simulink model "powerfrompropagatorLoLaSat"  (R2023b)
settings: Solver=FixedStepAuto  StartTime=0.0  StopTime=t_sim  FixedStep=TimeStep  RelTol=1e-3
undefined symbols (not defined in the file or in its folder): angle_roll, date, juliandate, MODE, Psa_X, Psa_Y, PsaX, PsaY
libraries: dspmathops x16, vrlib x12, aerolibutil x9, sharedtransform x9, sharedutil x4
settings Model: Creator=colpari  LastModifiedBy=lricc
settings SolverCC: AlgebraicLoopSolver=TrustRegion
settings OptimizationCC: ReuseModelBlockBuffer=off
settings DebuggingCC: UnconnectedInputMsg=warning  UnconnectedOutputMsg=warning  UnconnectedLineMsg=warning
settings ModelReferenceCC: EnableRefExpFcnMdlSchedulingChecks=on
settings RTWCC: DLArmComputeVersion=19.05

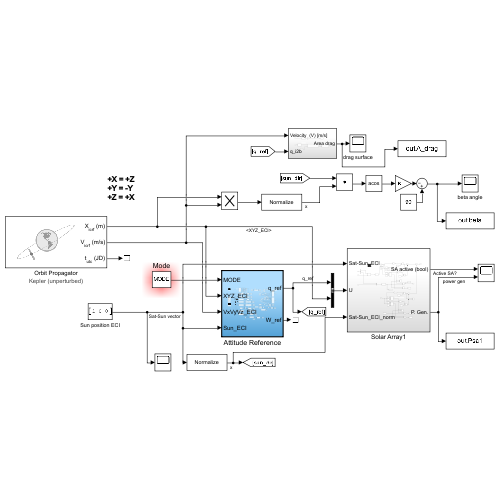
[thumbnail: Simulink's stored preview of the top-level diagram]
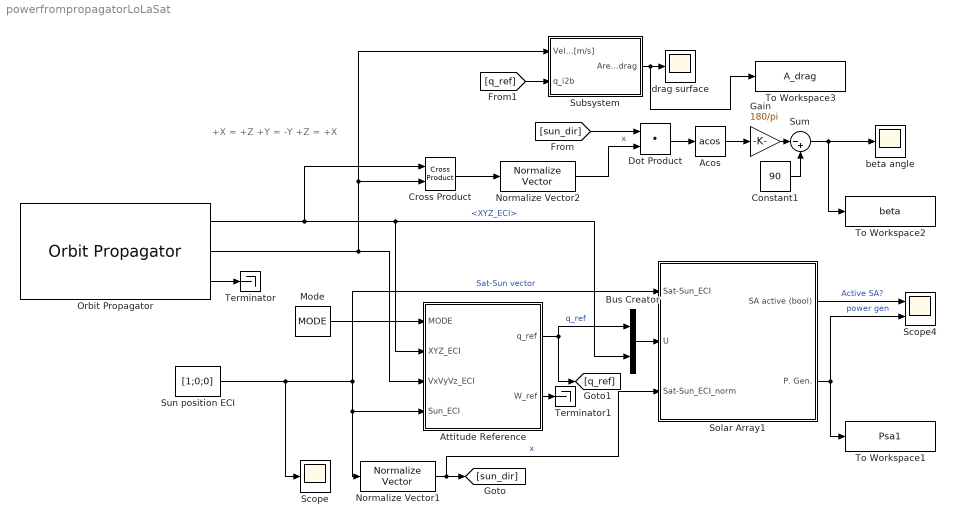
== system powerfrompropagatorLoLaSat ==
  note: +X = +Z
      | +Y = -Y
      | +Z = +X
  Acos : Trigonometry  Operator=acos
  Attitude Reference : Subsystem  TreatAsAtomicUnit=on
  Bus Creator : BusCreator  Inputs=2
  Constant1 : Constant  Value=90
  Cross Product : vrlib/Utilities/Cross Product
  Dot Product : DotProduct  OutDataTypeStr=Inherit: Inherit via internal rule
  Gain : Gain  Gain=180/pi
  Mode : Constant  Value=MODE  OutDataTypeStr=int8
  Normalize Vector1 : vrlib/Utilities/Normalize Vector  maxzero=0
  Normalize Vector2 : vrlib/Utilities/Normalize Vector  maxzero=0
  Orbit Propagator : OrbitPropagator  startDate=juliandate(date.year, date.month, date.day, date.hour, date.minutes, date.seconds)  semiMajorAxis=orbit.a  eccentricity=orbit.e  inclination=orbit.i  raan=orbit.O  argPeriapsis=orbit.o  trueAnomaly=orbit.nu  inertialPosition=[3649700.0 3308200.0 -4676600.0]  inertialVelocity=[-2750.8 6666.4 2573.4]  fixedPosition=[-4142689.0 -2676864.7 -4669861.6]  fixedVelocity=[1452.7 -6720.7 2568.1]  customR=3396200  customMu=4.305e13  customJ2=1.0826269e-03  customOmega=4.06125949e-3
      settings: AttributesFormatString=%<propagator>
  Scope : Scope
  Scope4 : Scope  NumInputPorts=2
  Solar Array1 : Subsystem
  Subsystem : Subsystem
  Sum : Sum  Inputs=|-+
  Sun position ECI : Constant  Value=[1;0;0]
  Terminator : Terminator
  Terminator1 : Terminator
  To Workspace1 : ToWorkspace  VariableName=Psa1  SaveFormat=Timeseries  SampleTime=-1
  To Workspace2 : ToWorkspace  VariableName=beta  SaveFormat=Timeseries  SampleTime=-1
  To Workspace3 : ToWorkspace  VariableName=A_drag  SaveFormat=Timeseries  SampleTime=-1
  beta angle : Scope
  drag surface : Scope
  wires:
  Dot Product/1 -> Acos/1
  Attitude Reference/1(q_ref) -> [q_ref], Bus Creator/1  "q_ref"
  Sum/1 -> beta angle/1, To Workspace2/1
  Cross Product/1 -> Normalize Vector2/1
  Solar Array1/2(P. Gen.) -> To Workspace1/1, Scope4/2  "power gen"
  [sun_dir] -> Dot Product/1
  Acos/1 -> Gain/1
  Orbit Propagator/2 -> Attitude Reference/3(VxVyVz_ECI), Subsystem/1(Velocity  (V) [m/s]), Cross Product/2
  Gain/1 -> Sum/1
  Sun position ECI/1 -> Scope/1, Solar Array1/1(Sat-Sun_ECI), Attitude Reference/4(Sun_ECI), Normalize Vector1/1  "Sat-Sun vector"
  Constant1/1 -> Sum/2
  Normalize Vector1/1 -> Solar Array1/3(Sat-Sun_ECI_norm), [sun_dir]  "x"
  Bus Creator/1 -> Solar Array1/2(U)
  Normalize Vector2/1 -> Dot Product/2  "x"
  Solar Array1/1(SA active (bool)) -> Scope4/1  "Active SA?"
  Orbit Propagator/1 -> Attitude Reference/2(XYZ_ECI), Bus Creator/2, Cross Product/1  "<XYZ_ECI>"
  Orbit Propagator/3 -> Terminator/1
  Attitude Reference/2(W_ref) -> Terminator1/1
  Mode/1 -> Attitude Reference/1(MODE)
  [q_ref] -> Subsystem/2(q_i2b)
  Subsystem/1(Area drag) -> To Workspace3/1, drag surface/1

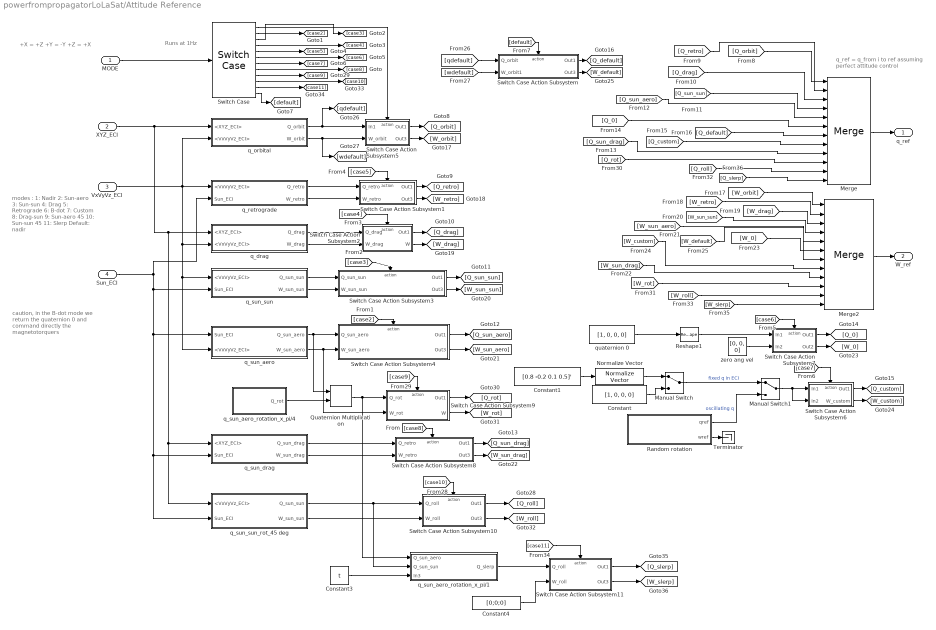
== system powerfrompropagatorLoLaSat/Attitude Reference ==
  note: caution, in the B-dot mode we return the quaternion 0 and command directly the magnetotorquers
  note: modes :
      | 1: Nadir
      | 2: Sun-aero
      | 3: Sun-sun
      | 4: Drag
      | 5: Retrograde
      | 6: B-dot
      | 7: Custom
      | 8: Drag-sun
      | 9: Sun-aero 45
      | 10: Sun-sun 45
      | 11: Slerp
      | Default: nadir
  note: q_ref  = q_from i to ref
      | assuming perfect attitude control
  note: Runs at 1Hz
  note: +X = +Z
      | +Y = -Y
      | +Z = +X
  MODE : Inport  OutMin=1  OutMax=100  OutDataTypeStr=int8
  XYZ_ECI : Inport  Port=2
  VxVyVz_ECI : Inport  Port=3
  Sun_ECI : Inport  Port=4
  Constant : Constant  Value=[1, 0, 0, 0]
  Constant1 : Constant  Value=[0.8 -0.2 0.1 0.5]'
  Constant3 : Constant  Value=t
  Constant4 : Constant  Value=[0;0;0]
  Manual Switch : ManualSwitch
  Manual Switch1 : ManualSwitch
  Merge : Merge  Inputs=12
  Merge2 : Merge  Inputs=12
  Normalize Vector : vrlib/Utilities/Normalize Vector  maxzero=0
  Quaternion Multiplication : aerolibutil/Quaternion Multiplication
  Random rotation : Subsystem
  Reshape1 : Reshape  OutputDimensionality=Column vector (2-D)
  Switch Case : SwitchCase  CaseConditions={1, 2, 3, 4, 5, 6, 7, 8, 9, 10, 11}
  Switch Case Action Subsystem : Subsystem  TreatAsAtomicUnit=on
  Switch Case Action Subsystem1 : Subsystem  TreatAsAtomicUnit=on
  Switch Case Action Subsystem10 : Subsystem  TreatAsAtomicUnit=on
  Switch Case Action Subsystem11 : Subsystem  TreatAsAtomicUnit=on
  Switch Case Action Subsystem2 : Subsystem  TreatAsAtomicUnit=on
  Switch Case Action Subsystem3 : Subsystem  TreatAsAtomicUnit=on
  Switch Case Action Subsystem4 : Subsystem  TreatAsAtomicUnit=on
  Switch Case Action Subsystem5 : Subsystem  TreatAsAtomicUnit=on
  Switch Case Action Subsystem6 : Subsystem  TreatAsAtomicUnit=on
  Switch Case Action Subsystem7 : Subsystem  TreatAsAtomicUnit=on
  Switch Case Action Subsystem8 : Subsystem  TreatAsAtomicUnit=on
  Switch Case Action Subsystem9 : Subsystem  TreatAsAtomicUnit=on
  Terminator : Terminator
  q_drag : Subsystem
  q_orbital : Subsystem
  q_retrograde : Subsystem
  q_sun_aero : Subsystem
  q_sun_aero_rotation_x_pi/1 : Subsystem
  q_sun_aero_rotation_x_pi/4 : Subsystem
  q_sun_drag : Subsystem
  q_sun_sun : Subsystem
  q_sun_sun_rot_45 deg : Subsystem
  quaternion 0 : Constant  Value=[1, 0, 0, 0]
  zero ang vel : Constant  Value=[0, 0, 0]
  q_ref : Outport  VectorParamsAs1DForOutWhenUnconnected=off
  W_ref : Outport  Port=2
  wires:
  quaternion 0/1 -> Reshape1/1
  Reshape1/1 -> Switch Case Action Subsystem7/1(In1)
  Constant/1 -> Manual Switch/2
  Constant1/1 -> Normalize Vector/1
  Normalize Vector/1 -> Manual Switch/1
  zero ang vel/1 -> Switch Case Action Subsystem7/2(In2)
  Manual Switch/1 -> Manual Switch1/1  "fixed q in ECI"
  Random rotation/1(qref) -> Manual Switch1/2  "oscillating q"
  Manual Switch1/1 -> Switch Case Action Subsystem6/2(In2), Switch Case Action Subsystem6/1(In1)
  [default] -> Switch Case Action Subsystem/Action
  Switch Case/7 -> [case7]
  Switch Case/4 -> [case4]
  Switch Case/5 -> [case5]
  [case3] -> Switch Case Action Subsystem3/Action
  [case5] -> Switch Case Action Subsystem1/Action
  Switch Case/3 -> [case3]
  Switch Case/2 -> [case2]
  q_drag/2(W_drag) -> Switch Case Action Subsystem2/2(W_drag)
  q_sun_drag/2(W_sun_drag) -> Switch Case Action Subsystem8/2(W_retro)
  q_sun_aero/2(W_sun_aero) -> Switch Case Action Subsystem9/2(W_rot), Switch Case Action Subsystem4/2(W_sun_aero)
  Switch Case/1 -> Switch Case Action Subsystem5/Action
  [case8] -> Switch Case Action Subsystem8/Action
  Switch Case/8 -> [case8]
  q_drag/1(Q_drag) -> Switch Case Action Subsystem2/1(Q_drag)
  Switch Case/12 -> [default]
  q_sun_sun/2(W_sun_sun) -> Switch Case Action Subsystem3/2(W_sun_sun)
  q_retrograde/2(W_retro) -> Switch Case Action Subsystem1/2(W_retro)
  q_sun_sun/1(Q_sun_sun) -> Switch Case Action Subsystem3/1(Q_sun_sun)
  q_sun_aero/1(Q_sun_aero) -> Quaternion Multiplication/1, Switch Case Action Subsystem4/1(Q_sun_aero)
  q_sun_drag/1(Q_sun_drag) -> Switch Case Action Subsystem8/1(Q_retro)
  Merge2/1 -> W_ref/1
  [case2] -> Switch Case Action Subsystem4/Action
  [case4] -> Switch Case Action Subsystem2/Action
  q_orbital/1(Q_orbit) -> [qdefault], Switch Case Action Subsystem5/1(In1)
  q_retrograde/1(Q_retro) -> Switch Case Action Subsystem1/1(Q_retro)
  q_orbital/2(W_orbit) -> [wdefault], Switch Case Action Subsystem5/2(W_orbit)
  Switch Case/6 -> [case6]
  VxVyVz_ECI/1 -> q_orbital/2(<VxVyVz_ECI>), q_retrograde/1(<VxVyVz_ECI>), q_drag/2(<VxVyVz_ECI>), q_sun_aero/2(<VxVyVz_ECI>), q_sun_sun/1(<VxVyVz_ECI>)
  Merge/1 -> q_ref/1
  MODE/1 -> Switch Case/1
  Random rotation/2(wref) -> Terminator/1
  [case6] -> Switch Case Action Subsystem7/Action
  [case7] -> Switch Case Action Subsystem6/Action
  Switch Case Action Subsystem5/1(Out1) -> [Q_orbit]
  [Q_orbit] -> Merge/1
  Switch Case Action Subsystem1/1(Out1) -> [Q_retro]
  [Q_retro] -> Merge/2
  Switch Case Action Subsystem2/1(Out1) -> [Q_drag]
  [Q_drag] -> Merge/3
  Switch Case Action Subsystem3/1(Out1) -> [Q_sun_sun]
  [Q_sun_sun] -> Merge/4
  Switch Case Action Subsystem4/1(Out1) -> [Q_sun_aero]
  [Q_sun_aero] -> Merge/5
  Switch Case Action Subsystem8/1(Out1) -> [Q_sun_drag]
  [Q_sun_drag] -> Merge/9
  Switch Case Action Subsystem7/1(Out1) -> [Q_0]
  [Q_0] -> Merge/6
  Switch Case Action Subsystem6/1(Out1) -> [Q_custom]
  [Q_custom] -> Merge/8
  Switch Case Action Subsystem/1(Out1) -> [Q_default]
  [Q_default] -> Merge/7
  Switch Case Action Subsystem5/2(Out3) -> [W_orbit]
  [W_orbit] -> Merge2/1
  Switch Case Action Subsystem1/2(Out3) -> [W_retro]
  [W_retro] -> Merge2/2
  Switch Case Action Subsystem2/2(W) -> [W_drag]
  [W_drag] -> Merge2/3
  Switch Case Action Subsystem3/2(Out3) -> [W_sun_sun]
  [W_sun_sun] -> Merge2/4
  Switch Case Action Subsystem4/2(Out3) -> [W_sun_aero]
  [W_sun_aero] -> Merge2/5
  Switch Case Action Subsystem8/2(Out3) -> [W_sun_drag]
  [W_sun_drag] -> Merge2/9
  Switch Case Action Subsystem7/2(Out2) -> [W_0]
  [W_0] -> Merge2/6
  Switch Case Action Subsystem6/2(W_custom) -> [W_custom]
  [W_custom] -> Merge2/8
  Switch Case Action Subsystem/2(Out3) -> [W_default]
  [W_default] -> Merge2/7
  [qdefault] -> Switch Case Action Subsystem/1(Q_orbit)
  [wdefault] -> Switch Case Action Subsystem/2(W_orbit1)
  q_sun_aero_rotation_x_pi/4/1(Q_rot) -> Quaternion Multiplication/2
  Quaternion Multiplication/1 -> q_sun_aero_rotation_x_pi/1/1(Q_sun_aero), Switch Case Action Subsystem9/1(Q_rot)
  Switch Case/9 -> [case9]
  [case9] -> Switch Case Action Subsystem9/Action
  Switch Case Action Subsystem9/1(Out1) -> [Q_rot]
  Switch Case Action Subsystem9/2(W) -> [W_rot]
  [Q_rot] -> Merge/10
  [W_rot] -> Merge2/10
  Sun_ECI/1 -> q_retrograde/2(Sun_ECI), q_sun_sun_rot_45 deg/2(Sun_ECI), q_sun_drag/2(Sun_ECI), q_sun_aero/1(Sun_ECI), q_sun_sun/2(Sun_ECI)
  q_sun_sun_rot_45 deg/1(Q_sun_sun) -> q_sun_aero_rotation_x_pi/1/2(Q_sun_sun), Switch Case Action Subsystem10/1(Q_roll)
  XYZ_ECI/1 -> q_sun_drag/1(<XYZ_ECI>), q_sun_sun_rot_45 deg/1(<VxVyVz_ECI>), q_drag/1(<XYZ_ECI>), q_orbital/1(<XYZ_ECI>)
  Switch Case Action Subsystem10/1(Out1) -> [Q_roll]
  [case10] -> Switch Case Action Subsystem10/Action
  q_sun_sun_rot_45 deg/2(W_sun_sun) -> Switch Case Action Subsystem10/2(W_roll)
  Switch Case Action Subsystem10/2(Out3) -> [W_roll]
  Switch Case/10 -> [case10]
  [Q_roll] -> Merge/11
  [W_roll] -> Merge2/11
  Switch Case/11 -> [case11]
  [W_slerp] -> Merge2/12
  Constant3/1 -> q_sun_aero_rotation_x_pi/1/3(In3)
  Switch Case Action Subsystem11/2(Out3) -> [W_slerp]
  [case11] -> Switch Case Action Subsystem11/Action
  Switch Case Action Subsystem11/1(Out1) -> [Q_slerp]
  q_sun_aero_rotation_x_pi/1/1(Q_slerp) -> Switch Case Action Subsystem11/1(Q_roll)
  Constant4/1 -> Switch Case Action Subsystem11/2(W_roll)
  [Q_slerp] -> Merge/12

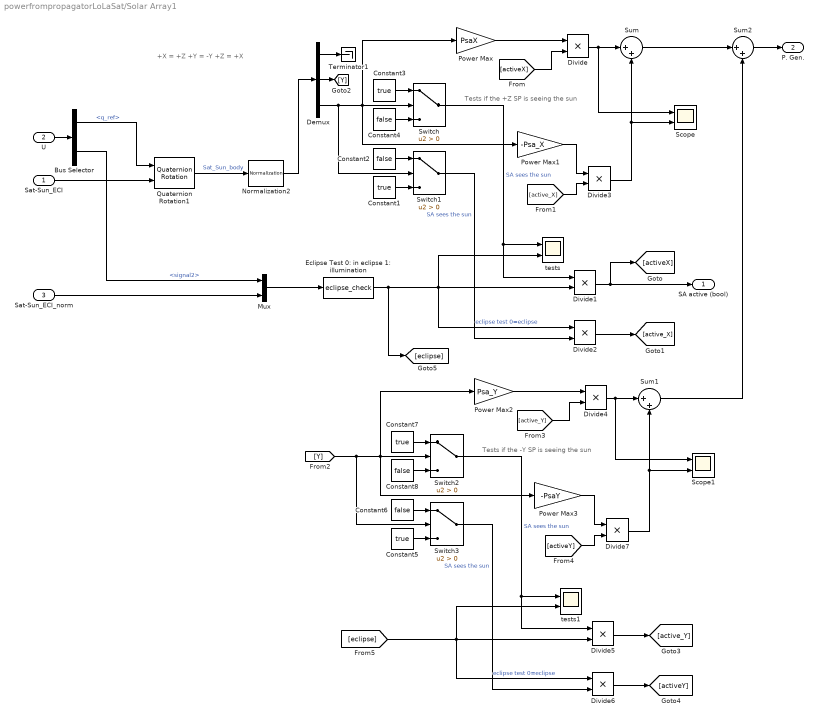
== system powerfrompropagatorLoLaSat/Solar Array1 ==
  note: Tests if the +Z SP is seeing the sun
  note: +X = +Z
      | +Y = -Y
      | +Z = +X
  note: Tests if the -Y SP is seeing the sun
  Sat-Sun_ECI : Inport
  U : Inport  Port=2
  Sat-Sun_ECI_norm : Inport  Port=3
  Bus Selector : BusSelector  OutputSignals=q_ref,signal2
  Constant{1,3,5,7} (4 alike) : Constant  Value=true
  Constant{2,4,6,8} (4 alike) : Constant  Value=false
  Demux : Demux  Outputs=3
  Divide{,1..7} (8 alike) : Product  Inputs=**
  Eclipse Test 0: in eclipse 1: illumination : MATLABFcn  MATLABFcn=eclipse_check
  Mux : Mux  Inputs=2
  Normalization2 : dspmathops/Normalization  NormType=2-norm  Bias=1e-10  NormOver=Each column  Dimension=1  roundingMode=Floor  overflowMode=off  accumDataTypeStr=Inherit: Same as product output  accumLastDataTypeStr=Inherit: Same as product output  outputDataTypeStr=Inherit: Same as product output  outputMin=[]  outputMax=[]  outputLastDataTypeStr=Inherit: Same as product output
  Power Max : Gain  Gain=PsaX
  Power Max1 : Gain  Gain=-Psa_X
  Power Max2 : Gain  Gain=Psa_Y
  Power Max3 : Gain  Gain=-PsaY
  Quaternion Rotation1 : aerolibutil/Quaternion Rotation
  Scope : Scope  NumInputPorts=2
  Scope1 : Scope  NumInputPorts=2
  Sum : Sum  Inputs=|++
  Sum1 : Sum  Inputs=|++
  Sum2 : Sum  Inputs=|++
  Switch{,1..3} (4 alike) : Switch  Criteria=u2 > Threshold  SaturateOnIntegerOverflow=off  InputSameDT=off
  Terminator1 : Terminator
  tests : Scope  NumInputPorts=2
  tests1 : Scope  NumInputPorts=2
  SA active (bool) : Outport  VectorParamsAs1DForOutWhenUnconnected=off
  P. Gen. : Outport  Port=2
  wires:
  Switch/1 -> Divide1/1, tests/1  "SA sees the sun"
  U/1 -> Bus Selector/1
  Bus Selector/1 -> Quaternion Rotation1/1  "<q_ref>"
  Quaternion Rotation1/1 -> Normalization2/1  "Sat_Sun_body"
  Constant3/1 -> Switch/1
  Demux/2 -> [Y]
  Demux/1 -> Terminator1/1
  Bus Selector/2 -> Mux/1  "<signal2>"
  Divide1/1 -> [activeX], SA active (bool)/1
  Constant4/1 -> Switch/3
  Normalization2/1 -> Demux/1
  Divide/1 -> Scope/1, Sum/1
  Power Max/1 -> Divide/1
  [activeX] -> Divide/2
  Sat-Sun_ECI_norm/1 -> Mux/2
  Mux/1 -> Eclipse Test 0: in eclipse 1: illumination/1
  Eclipse Test 0: in eclipse 1: illumination/1 -> [eclipse], Divide2/1, tests/2, Divide1/2  "eclipse test 0=eclipse"
  Demux/3 -> Switch1/2, Power Max1/1, Power Max/1, Switch/2
  Constant2/1 -> Switch1/1
  Constant1/1 -> Switch1/3
  Switch1/1 -> Divide2/2  "SA sees the sun"
  Divide2/1 -> [active_X]
  [active_X] -> Divide3/2
  Power Max1/1 -> Divide3/1
  Divide3/1 -> Sum/2, Scope/2
  Sum/1 -> Sum2/1
  [Y] -> Switch3/2, Power Max3/1, Power Max2/1, Switch2/2
  [eclipse] -> Divide6/1, tests1/2, Divide5/2  "eclipse test 0=eclipse"
  [active_Y] -> Divide4/2
  Constant7/1 -> Switch2/1
  Divide5/1 -> [active_Y]
  Constant8/1 -> Switch2/3
  Switch2/1 -> Divide5/1, tests1/1  "SA sees the sun"
  Sum1/1 -> Sum2/2
  Divide6/1 -> [activeY]
  Divide4/1 -> Scope1/1, Sum1/1
  Switch3/1 -> Divide6/2  "SA sees the sun"
  Constant6/1 -> Switch3/1
  Power Max2/1 -> Divide4/1
  [activeY] -> Divide7/2
  Power Max3/1 -> Divide7/1
  Divide7/1 -> Scope1/2, Sum1/2
  Constant5/1 -> Switch3/3
  Sum2/1 -> P. Gen./1
  Sat-Sun_ECI/1 -> Quaternion Rotation1/2

== system powerfrompropagatorLoLaSat/Subsystem ==
  note: wind unit vector [ECI]
  note: ECI to body
  Velocity  (V) [m/s] : Inport
  q_i2b : Inport  Port=2
  Calculate - Az & El Angle : Subsystem
  Gain2 : Gain
  Lookup - Area Drag : Lookup2D  RowIndex=LLSataero.Az  ColumnIndex=LLSataero.El  Table=LLSataero.A_drag'  SaturateOnIntegerOverflow=off  InputSameDT=off
  Quaternions to Direction Cosine Matrix : sharedtransform/Quaternions to  Direction Cosine Matrix  aMode=aMode
  Vector Normal : vrlib/Utilities/Normalize Vector  maxzero=0
  Area drag : Outport
  wires:
  Lookup - Area Drag/1 -> Area drag/1
  Calculate - Az & El Angle/2(Az) -> Lookup - Area Drag/2
  Calculate - Az & El Angle/1(El) -> Lookup - Area Drag/1
  Vector Normal/1 -> Gain2/1
  Velocity  (V) [m/s]/1 -> Vector Normal/1
  Gain2/1 -> [u_wind]
  [u_wind] -> Calculate - Az & El Angle/2(Wind unit ECI)
  Quaternions to Direction Cosine Matrix/1 -> Calculate - Az & El Angle/1(attitude)
  q_i2b/1 -> Quaternions to Direction Cosine Matrix/1

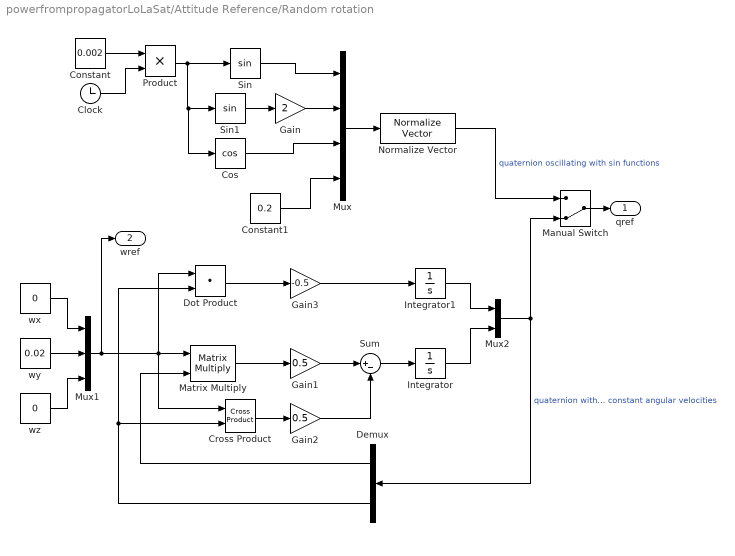
== system powerfrompropagatorLoLaSat/Attitude Reference/Random rotation ==
  Clock : Clock
      settings: Decimation=TimeStep
  Constant : Constant  Value=0.002
  Constant1 : Constant  Value=0.2
  Cos : Trigonometry  Operator=cos
  Cross Product : vrlib/Utilities/Cross Product
  Demux : Demux  Outputs=[1;3]
  Dot Product : DotProduct  OutDataTypeStr=Inherit: Inherit via internal rule
  Gain : Gain  Gain=2
  Gain1 : Gain  Gain=0.5
  Gain2 : Gain  Gain=0.5
  Gain3 : Gain  Gain=-0.5
  Integrator : Integrator  InitialCondition=[0;0;0]
  Integrator1 : Integrator  InitialCondition=1
  Manual Switch : ManualSwitch  CurrentSetting=0
  Matrix Multiply : Product  Multiplication=Matrix(*)
  Mux : Mux
  Mux1 : Mux  Inputs=3
  Mux2 : Mux  Inputs=[1;3]
  Normalize Vector : vrlib/Utilities/Normalize Vector  maxzero=0
  Product : Product
  Sin : Trigonometry
  Sin1 : Trigonometry
  Sum : Sum  Inputs=|+-
  wx : Constant  Value=0
  wy : Constant  Value=0.02
  wz : Constant  Value=0
  qref : Outport
  wref : Outport  Port=2
  wires:
  Mux/1 -> Normalize Vector/1
  Normalize Vector/1 -> Manual Switch/1  "quaternion oscillating with sin functions"
  Constant/1 -> Product/1
  Clock/1 -> Product/2
  Product/1 -> Cos/1, Sin1/1, Sin/1
  Sin/1 -> Mux/1
  Sin1/1 -> Gain/1
  Gain/1 -> Mux/2
  Cos/1 -> Mux/3
  Constant1/1 -> Mux/4
  Manual Switch/1 -> qref/1
  wx/1 -> Mux1/1
  wy/1 -> Mux1/2
  wz/1 -> Mux1/3
  Mux1/1 -> wref/1, Dot Product/1, Cross Product/1, Matrix Multiply/1
  Matrix Multiply/1 -> Gain1/1
  Gain1/1 -> Sum/1
  Sum/1 -> Integrator/1
  Integrator/1 -> Mux2/2
  Mux2/1 -> Demux/1, Manual Switch/2  "quaternion with constant angular velocities"
  Demux/1 -> Matrix Multiply/2
  Cross Product/1 -> Gain2/1
  Gain2/1 -> Sum/2
  Dot Product/1 -> Gain3/1
  Gain3/1 -> Integrator1/1
  Integrator1/1 -> Mux2/1
  Demux/2 -> Cross Product/2, Dot Product/2

== system powerfrompropagatorLoLaSat/Attitude Reference/Switch Case Action Subsystem ==
  Q_orbit : Inport
  W_orbit1 : Inport  Port=2
  Action Port : ActionPort  ActionPortLabel=default:
  Out1 : Outport  VectorParamsAs1DForOutWhenUnconnected=off
  Out3 : Outport  Port=2  VectorParamsAs1DForOutWhenUnconnected=off
  wires:
  Q_orbit/1 -> Out1/1
  W_orbit1/1 -> Out3/1

== system powerfrompropagatorLoLaSat/Attitude Reference/Switch Case Action Subsystem1 ==
  Q_retro : Inport
  W_retro : Inport  Port=2
  Action Port : ActionPort  ActionPortLabel=case [ 5 ]:
  Out1 : Outport  VectorParamsAs1DForOutWhenUnconnected=off
  Out3 : Outport  Port=2  VectorParamsAs1DForOutWhenUnconnected=off
  wires:
  Q_retro/1 -> Out1/1
  W_retro/1 -> Out3/1

== system powerfrompropagatorLoLaSat/Attitude Reference/Switch Case Action Subsystem10 ==
  note: from I to SS
  Q_roll : Inport
  W_roll : Inport  Port=2
  Action Port : ActionPort  ActionPortLabel=case [ 10 ]:
  Out1 : Outport  VectorParamsAs1DForOutWhenUnconnected=off
  Out3 : Outport  Port=2  VectorParamsAs1DForOutWhenUnconnected=off
  wires:
  Q_roll/1 -> Out1/1
  W_roll/1 -> Out3/1

== system powerfrompropagatorLoLaSat/Attitude Reference/Switch Case Action Subsystem11 ==
  note: from I to SS
  Q_roll : Inport
  W_roll : Inport  Port=2
  Action Port : ActionPort  ActionPortLabel=case [ 11 ]:
  Out1 : Outport  VectorParamsAs1DForOutWhenUnconnected=off
  Out3 : Outport  Port=2  VectorParamsAs1DForOutWhenUnconnected=off
  wires:
  Q_roll/1 -> Out1/1
  W_roll/1 -> Out3/1

== system powerfrompropagatorLoLaSat/Attitude Reference/Switch Case Action Subsystem2 ==
  note: q from I to O + rotation
  Q_drag : Inport
  W_drag : Inport  Port=2
  Action Port : ActionPort  ActionPortLabel=case [ 4 ]:
  Out1 : Outport  VectorParamsAs1DForOutWhenUnconnected=off
  W : Outport  Port=2
  wires:
  Q_drag/1 -> Out1/1
  W_drag/1 -> W/1

== system powerfrompropagatorLoLaSat/Attitude Reference/Switch Case Action Subsystem3 ==
  Q_sun_sun : Inport
  W_sun_sun : Inport  Port=2
  Action Port : ActionPort  ActionPortLabel=case [ 3 ]:
  Out1 : Outport  VectorParamsAs1DForOutWhenUnconnected=off
  Out3 : Outport  Port=2  VectorParamsAs1DForOutWhenUnconnected=off
  wires:
  Q_sun_sun/1 -> Out1/1
  W_sun_sun/1 -> Out3/1

== system powerfrompropagatorLoLaSat/Attitude Reference/Switch Case Action Subsystem4 ==
  Q_sun_aero : Inport
  W_sun_aero : Inport  Port=2
  Action Port : ActionPort  ActionPortLabel=case [ 2 ]:
  Out1 : Outport  VectorParamsAs1DForOutWhenUnconnected=off
  Out3 : Outport  Port=2  VectorParamsAs1DForOutWhenUnconnected=off
  wires:
  Q_sun_aero/1 -> Out1/1
  W_sun_aero/1 -> Out3/1

== system powerfrompropagatorLoLaSat/Attitude Reference/Switch Case Action Subsystem5 ==
  In1 : Inport
  W_orbit : Inport  Port=2
  Action Port : ActionPort  ActionPortLabel=case [ 1 ]:
  Out1 : Outport  VectorParamsAs1DForOutWhenUnconnected=off
  Out3 : Outport  Port=2  VectorParamsAs1DForOutWhenUnconnected=off
  wires:
  In1/1 -> Out1/1
  W_orbit/1 -> Out3/1

== system powerfrompropagatorLoLaSat/Attitude Reference/Switch Case Action Subsystem6 ==
  In1 : Inport
  In2 : Inport  Port=2
  Action Port : ActionPort  ActionPortLabel=case [ 7 ]:
  Derivative : Derivative
  Matrix Multiply : Product  Multiplication=Matrix(*)
  Quaternions to Direction Cosine Matrix : sharedtransform/Quaternions to  Direction Cosine Matrix  aMode=aMode
  Transpose : Math  Operator=transpose
  Transpose1 : Math  Operator=transpose
  gets vector from Skew Matrix : MATLABFcn  MATLABFcn=vec_from_skew
  Out1 : Outport  VectorParamsAs1DForOutWhenUnconnected=off
  W_custom : Outport  Port=2
  wires:
  In1/1 -> Out1/1
  In2/1 -> Quaternions to Direction Cosine Matrix/1
  Quaternions to Direction Cosine Matrix/1 -> Transpose1/1
  Matrix Multiply/1 -> gets vector from Skew Matrix/1
  Transpose/1 -> Derivative/1
  gets vector from Skew Matrix/1 -> W_custom/1
  Derivative/1 -> Matrix Multiply/1
  Transpose1/1 -> Transpose/1, Matrix Multiply/2

== system powerfrompropagatorLoLaSat/Attitude Reference/Switch Case Action Subsystem7 ==
  In1 : Inport
  In2 : Inport  Port=2
  Action Port : ActionPort  ActionPortLabel=case [ 6 ]:
  Out1 : Outport  VectorParamsAs1DForOutWhenUnconnected=off
  Out2 : Outport  Port=2  VectorParamsAs1DForOutWhenUnconnected=off
  wires:
  In1/1 -> Out1/1
  In2/1 -> Out2/1

== system powerfrompropagatorLoLaSat/Attitude Reference/Switch Case Action Subsystem8 ==
  Q_retro : Inport
  W_retro : Inport  Port=2
  Action Port : ActionPort  ActionPortLabel=case [ 8 ]:
  Out1 : Outport  VectorParamsAs1DForOutWhenUnconnected=off
  Out3 : Outport  Port=2  VectorParamsAs1DForOutWhenUnconnected=off
  wires:
  Q_retro/1 -> Out1/1
  W_retro/1 -> Out3/1

== system powerfrompropagatorLoLaSat/Attitude Reference/Switch Case Action Subsystem9 ==
  note: q from I to O + rotation
  Q_rot : Inport
  W_rot : Inport  Port=2
  Action Port : ActionPort  ActionPortLabel=case [ 9 ]:
  Out1 : Outport  VectorParamsAs1DForOutWhenUnconnected=off
  W : Outport  Port=2
  wires:
  Q_rot/1 -> Out1/1
  W_rot/1 -> W/1

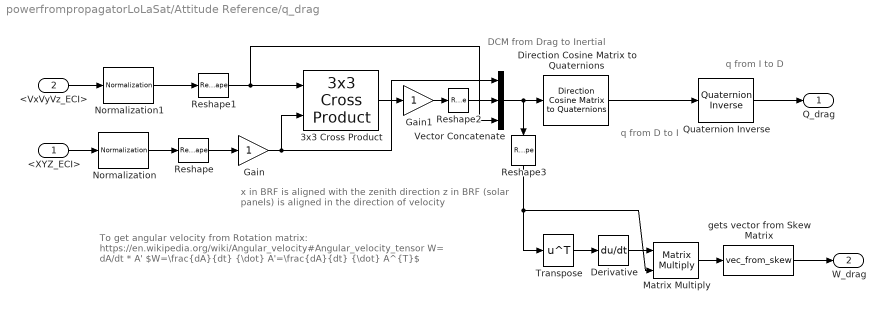
== system powerfrompropagatorLoLaSat/Attitude Reference/q_drag ==
  note: x in BRF is aligned with the zenith direction
      | z in BRF (solar panels) is aligned in the direction of velocity
  note: DCM from Drag to Inertial
  note: q from D to I
  note: q from I to D
  note: To get angular velocity from Rotation matrix:
      | https://en.wikipedia.org/wiki/Angular_velocity#Angular_velocity_tensor
      | W= dA/dt * A'
      | $W=\frac{dA}{dt} {\dot} A'=\frac{dA}{dt} {\dot} A^{T}$
  <XYZ_ECI> : Inport
  <VxVyVz_ECI> : Inport  Port=2
  3x3 Cross Product : sharedutil/3x3 Cross Product  aMode=aMode
  Derivative : Derivative
  Direction Cosine Matrix to Quaternions : sharedtransform/Direction Cosine Matrix  to Quaternions  aMode=0  action=None  tolerance=eps(2)
  Gain : Gain
  Gain1 : Gain
  Matrix Multiply : Product  Multiplication=Matrix(*)
  Normalization : dspmathops/Normalization  NormType=2-norm  Bias=1e-10  NormOver=Each column  Dimension=1  roundingMode=Floor  overflowMode=off  accumDataTypeStr=Inherit: Same as product output  accumLastDataTypeStr=Inherit: Same as product output  outputDataTypeStr=Inherit: Same as product output  outputMin=[]  outputMax=[]  outputLastDataTypeStr=Inherit: Same as product output
  Normalization1 : dspmathops/Normalization  NormType=2-norm  Bias=1e-10  NormOver=Each column  Dimension=1  roundingMode=Floor  overflowMode=off  accumDataTypeStr=Inherit: Same as product output  accumLastDataTypeStr=Inherit: Same as product output  outputDataTypeStr=Inherit: Same as product output  outputMin=[]  outputMax=[]  outputLastDataTypeStr=Inherit: Same as product output
  Quaternion Inverse : aerolibutil/Quaternion Inverse
  Reshape : Reshape  OutputDimensionality=Column vector (2-D)
  Reshape1 : Reshape  OutputDimensionality=Column vector (2-D)
  Reshape2 : Reshape  OutputDimensionality=Column vector (2-D)
  Reshape3 : Reshape  OutputDimensionality=Customize  OutputDimensions=[3,3]
  Transpose : Math  Operator=transpose
  Vector Concatenate : Concatenate  NumInputs=3  Mode=Multidimensional array  ConcatenateDimension=2
  gets vector from Skew Matrix : MATLABFcn  MATLABFcn=vec_from_skew
  Q_drag : Outport  VectorParamsAs1DForOutWhenUnconnected=off
  W_drag : Outport  Port=2
  wires:
  Normalization/1 -> Reshape/1
  Normalization1/1 -> Reshape1/1
  <VxVyVz_ECI>/1 -> Normalization1/1
  Reshape1/1 -> Vector Concatenate/3, 3x3 Cross Product/1
  <XYZ_ECI>/1 -> Normalization/1
  Reshape/1 -> Gain/1
  Gain/1 -> Vector Concatenate/1, 3x3 Cross Product/2
  Direction Cosine Matrix to Quaternions/1 -> Quaternion Inverse/1
  3x3 Cross Product/1 -> Gain1/1
  Gain1/1 -> Reshape2/1
  Quaternion Inverse/1 -> Q_drag/1
  Vector Concatenate/1 -> Reshape3/1, Direction Cosine Matrix to Quaternions/1
  gets vector from Skew Matrix/1 -> W_drag/1
  Matrix Multiply/1 -> gets vector from Skew Matrix/1
  Transpose/1 -> Derivative/1
  Derivative/1 -> Matrix Multiply/1
  Reshape2/1 -> Vector Concatenate/2
  Reshape3/1 -> Matrix Multiply/2, Transpose/1

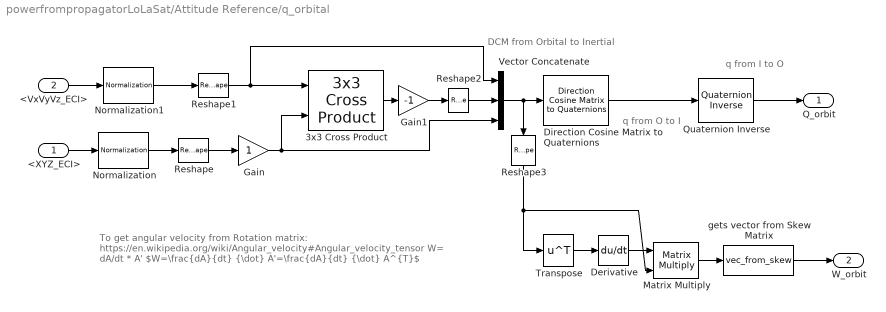
== system powerfrompropagatorLoLaSat/Attitude Reference/q_orbital ==
  note: DCM from Orbital to Inertial
  note: q from O to I
  note: q from I to O
  note: To get angular velocity from Rotation matrix:
      | https://en.wikipedia.org/wiki/Angular_velocity#Angular_velocity_tensor
      | W= dA/dt * A'
      | $W=\frac{dA}{dt} {\dot} A'=\frac{dA}{dt} {\dot} A^{T}$
  <XYZ_ECI> : Inport
  <VxVyVz_ECI> : Inport  Port=2
  3x3 Cross Product : sharedutil/3x3 Cross Product  aMode=aMode
  Derivative : Derivative
  Direction Cosine Matrix to Quaternions : sharedtransform/Direction Cosine Matrix  to Quaternions  aMode=0  action=None  tolerance=eps(2)
  Gain : Gain
  Gain1 : Gain  Gain=-1
  Matrix Multiply : Product  Multiplication=Matrix(*)
  Normalization : dspmathops/Normalization  NormType=2-norm  Bias=1e-10  NormOver=Each column  Dimension=1  roundingMode=Floor  overflowMode=off  accumDataTypeStr=Inherit: Same as product output  accumLastDataTypeStr=Inherit: Same as product output  outputDataTypeStr=Inherit: Same as product output  outputMin=[]  outputMax=[]  outputLastDataTypeStr=Inherit: Same as product output
  Normalization1 : dspmathops/Normalization  NormType=2-norm  Bias=1e-10  NormOver=Each column  Dimension=1  roundingMode=Floor  overflowMode=off  accumDataTypeStr=Inherit: Same as product output  accumLastDataTypeStr=Inherit: Same as product output  outputDataTypeStr=Inherit: Same as product output  outputMin=[]  outputMax=[]  outputLastDataTypeStr=Inherit: Same as product output
  Quaternion Inverse : aerolibutil/Quaternion Inverse
  Reshape : Reshape  OutputDimensionality=Column vector (2-D)
  Reshape1 : Reshape  OutputDimensionality=Column vector (2-D)
  Reshape2 : Reshape  OutputDimensionality=Column vector (2-D)
  Reshape3 : Reshape  OutputDimensionality=Customize  OutputDimensions=[3,3]
  Transpose : Math  Operator=transpose
  Vector Concatenate : Concatenate  NumInputs=3  Mode=Multidimensional array  ConcatenateDimension=2
  gets vector from Skew Matrix : MATLABFcn  MATLABFcn=vec_from_skew
  Q_orbit : Outport  VectorParamsAs1DForOutWhenUnconnected=off
  W_orbit : Outport  Port=2
  wires:
  Normalization/1 -> Reshape/1
  Normalization1/1 -> Reshape1/1
  <VxVyVz_ECI>/1 -> Normalization1/1
  Reshape1/1 -> 3x3 Cross Product/1, Vector Concatenate/1
  <XYZ_ECI>/1 -> Normalization/1
  Reshape/1 -> Gain/1
  Gain/1 -> 3x3 Cross Product/2, Vector Concatenate/3
  Direction Cosine Matrix to Quaternions/1 -> Quaternion Inverse/1
  3x3 Cross Product/1 -> Gain1/1
  Gain1/1 -> Reshape2/1
  Quaternion Inverse/1 -> Q_orbit/1
  Vector Concatenate/1 -> Reshape3/1, Direction Cosine Matrix to Quaternions/1
  gets vector from Skew Matrix/1 -> W_orbit/1
  Matrix Multiply/1 -> gets vector from Skew Matrix/1
  Transpose/1 -> Derivative/1
  Derivative/1 -> Matrix Multiply/1
  Reshape2/1 -> Vector Concatenate/2
  Reshape3/1 -> Matrix Multiply/2, Transpose/1

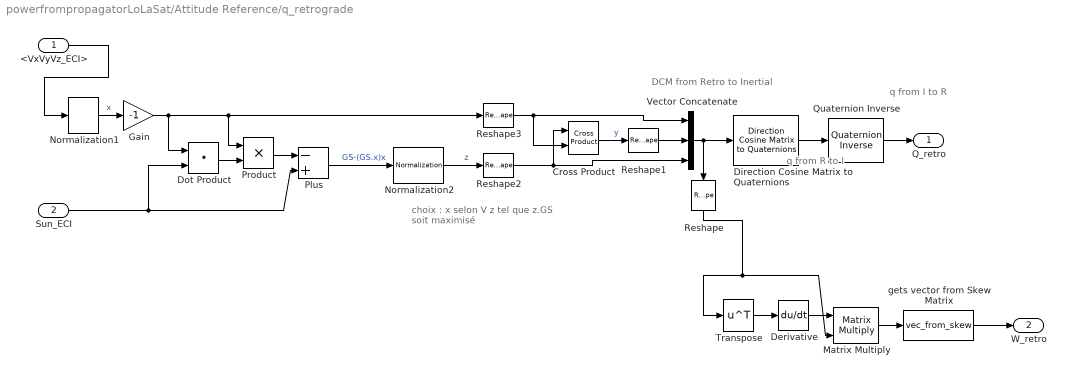
== system powerfrompropagatorLoLaSat/Attitude Reference/q_retrograde ==
  note: q from I to R
  note: q from R to I
  note: DCM from Retro to Inertial
  note: choix :
      | x selon V
      | z tel que z.GS soit maximisé
  <VxVyVz_ECI> : Inport
  Sun_ECI : Inport  Port=2
  Cross Product : vrlib/Utilities/Cross Product
  Derivative : Derivative
  Direction Cosine Matrix to Quaternions : sharedtransform/Direction Cosine Matrix  to Quaternions  aMode=0  action=None  tolerance=eps(2)
  Dot Product : DotProduct  OutDataTypeStr=Inherit: Inherit via internal rule
  Gain : Gain  Gain=-1
  Matrix Multiply : Product  Multiplication=Matrix(*)
  Normalization1 : dspmathops/Normalization  NormType=2-norm  Bias=1e-10  NormOver=Each column  Dimension=1  roundingMode=Floor  overflowMode=off  accumDataTypeStr=Inherit: Same as product output  accumLastDataTypeStr=Inherit: Same as product output  outputDataTypeStr=Inherit: Same as product output  outputMin=[]  outputMax=[]  outputLastDataTypeStr=Inherit: Same as product output
  Normalization2 : dspmathops/Normalization  NormType=2-norm  Bias=1e-10  NormOver=Each column  Dimension=1  roundingMode=Floor  overflowMode=off  accumDataTypeStr=Inherit: Same as product output  accumLastDataTypeStr=Inherit: Same as product output  outputDataTypeStr=Inherit: Same as product output  outputMin=[]  outputMax=[]  outputLastDataTypeStr=Inherit: Same as product output
  Plus : Sum  Inputs=-+
  Product : Product
  Quaternion Inverse : aerolibutil/Quaternion Inverse
  Reshape : Reshape  OutputDimensionality=Customize  OutputDimensions=[3,3]
  Reshape1 : Reshape  OutputDimensionality=Column vector (2-D)
  Reshape2 : Reshape  OutputDimensionality=Column vector (2-D)
  Reshape3 : Reshape  OutputDimensionality=Column vector (2-D)
  Transpose : Math  Operator=transpose
  Vector Concatenate : Concatenate  NumInputs=3  Mode=Multidimensional array  ConcatenateDimension=2
  gets vector from Skew Matrix : MATLABFcn  MATLABFcn=vec_from_skew
  Q_retro : Outport  VectorParamsAs1DForOutWhenUnconnected=off
  W_retro : Outport  Port=2
  wires:
  Quaternion Inverse/1 -> Q_retro/1
  Reshape2/1 -> Vector Concatenate/3, Cross Product/1
  Reshape3/1 -> Vector Concatenate/1, Cross Product/2
  Product/1 -> Plus/1
  Dot Product/1 -> Product/2
  Cross Product/1 -> Reshape1/1  "y"
  Normalization2/1 -> Reshape2/1  "z"
  Plus/1 -> Normalization2/1  "GS-(GS.x)x"
  Sun_ECI/1 -> Dot Product/2, Plus/2
  Direction Cosine Matrix to Quaternions/1 -> Quaternion Inverse/1
  Normalization1/1 -> Gain/1  "x"
  <VxVyVz_ECI>/1 -> Normalization1/1
  Reshape1/1 -> Vector Concatenate/2
  Gain/1 -> Dot Product/1, Product/1, Reshape3/1
  Vector Concatenate/1 -> Direction Cosine Matrix to Quaternions/1, Reshape/1
  gets vector from Skew Matrix/1 -> W_retro/1
  Matrix Multiply/1 -> gets vector from Skew Matrix/1
  Derivative/1 -> Matrix Multiply/1
  Transpose/1 -> Derivative/1
  Reshape/1 -> Transpose/1, Matrix Multiply/2

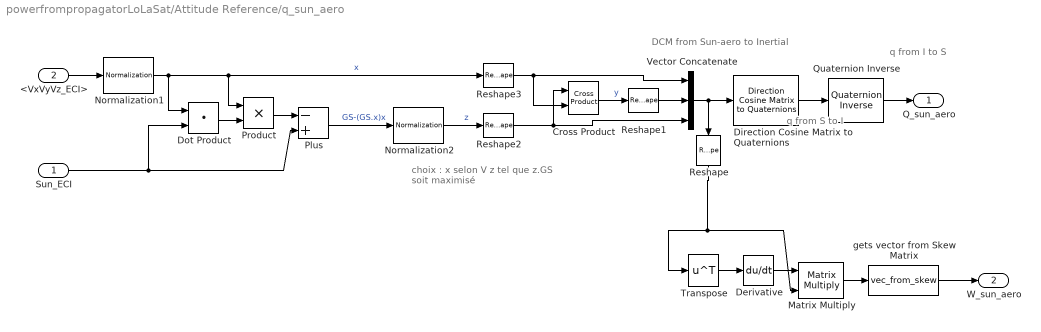
== system powerfrompropagatorLoLaSat/Attitude Reference/q_sun_aero ==
  note: q from I to S
  note: q from S to I
  note: DCM from Sun-aero to Inertial
  note: choix :
      | x selon V
      | z tel que z.GS soit maximisé
  Sun_ECI : Inport
  <VxVyVz_ECI> : Inport  Port=2
  Cross Product : vrlib/Utilities/Cross Product
  Derivative : Derivative
  Direction Cosine Matrix to Quaternions : sharedtransform/Direction Cosine Matrix  to Quaternions  aMode=0  action=None  tolerance=eps(2)
  Dot Product : DotProduct  OutDataTypeStr=Inherit: Inherit via internal rule
  Matrix Multiply : Product  Multiplication=Matrix(*)
  Normalization1 : dspmathops/Normalization  NormType=2-norm  Bias=1e-10  NormOver=Each column  Dimension=1  roundingMode=Floor  overflowMode=off  accumDataTypeStr=Inherit: Same as product output  accumLastDataTypeStr=Inherit: Same as product output  outputDataTypeStr=Inherit: Same as product output  outputMin=[]  outputMax=[]  outputLastDataTypeStr=Inherit: Same as product output
  Normalization2 : dspmathops/Normalization  NormType=2-norm  Bias=1e-10  NormOver=Each column  Dimension=1  roundingMode=Floor  overflowMode=off  accumDataTypeStr=Inherit: Same as product output  accumLastDataTypeStr=Inherit: Same as product output  outputDataTypeStr=Inherit: Same as product output  outputMin=[]  outputMax=[]  outputLastDataTypeStr=Inherit: Same as product output
  Plus : Sum  Inputs=-+
  Product : Product
  Quaternion Inverse : aerolibutil/Quaternion Inverse
  Reshape : Reshape  OutputDimensionality=Customize  OutputDimensions=[3,3]
  Reshape1 : Reshape  OutputDimensionality=Column vector (2-D)
  Reshape2 : Reshape  OutputDimensionality=Column vector (2-D)
  Reshape3 : Reshape  OutputDimensionality=Column vector (2-D)
  Transpose : Math  Operator=transpose
  Vector Concatenate : Concatenate  NumInputs=3  Mode=Multidimensional array  ConcatenateDimension=2
  gets vector from Skew Matrix : MATLABFcn  MATLABFcn=vec_from_skew
  Q_sun_aero : Outport  VectorParamsAs1DForOutWhenUnconnected=off
  W_sun_aero : Outport  Port=2
  wires:
  Quaternion Inverse/1 -> Q_sun_aero/1
  Reshape2/1 -> Vector Concatenate/3, Cross Product/1
  Reshape3/1 -> Vector Concatenate/1, Cross Product/2
  Product/1 -> Plus/1
  Dot Product/1 -> Product/2
  Cross Product/1 -> Reshape1/1  "y"
  Normalization2/1 -> Reshape2/1  "z"
  Plus/1 -> Normalization2/1  "GS-(GS.x)x"
  Sun_ECI/1 -> Dot Product/2, Plus/2
  Direction Cosine Matrix to Quaternions/1 -> Quaternion Inverse/1
  Normalization1/1 -> Dot Product/1, Product/1, Reshape3/1  "x"
  <VxVyVz_ECI>/1 -> Normalization1/1
  Reshape1/1 -> Vector Concatenate/2
  Transpose/1 -> Derivative/1
  Matrix Multiply/1 -> gets vector from Skew Matrix/1
  Derivative/1 -> Matrix Multiply/1
  Vector Concatenate/1 -> Direction Cosine Matrix to Quaternions/1, Reshape/1
  gets vector from Skew Matrix/1 -> W_sun_aero/1
  Reshape/1 -> Transpose/1, Matrix Multiply/2

== system powerfrompropagatorLoLaSat/Attitude Reference/q_sun_aero_rotation_x_pi//1 ==
  Q_sun_aero : Inport
  Q_sun_sun : Inport  Port=2
  In3 : Inport  Port=3
  Quaternion Interpolation : QuatInterp
  Quaternion Normalize : sharedutil/Quaternion Normalize  aMode=aMode
  Quaternion Normalize1 : sharedutil/Quaternion Normalize  aMode=aMode
  Q_slerp : Outport  VectorParamsAs1DForOutWhenUnconnected=off
  wires:
  Quaternion Interpolation/1 -> Q_slerp/1
  Q_sun_sun/1 -> Quaternion Normalize1/1
  Q_sun_aero/1 -> Quaternion Normalize/1
  In3/1 -> Quaternion Interpolation/3
  Quaternion Normalize/1 -> Quaternion Interpolation/1
  Quaternion Normalize1/1 -> Quaternion Interpolation/2

== system powerfrompropagatorLoLaSat/Attitude Reference/q_sun_aero_rotation_x_pi//4 ==
  Constant : Constant  Value=[1;0;0]
  Product : Product
  Reshape1 : Reshape  OutputDimensionality=Column vector (2-D)
  Vector Concatenate1 : Concatenate  Mode=Multidimensional array
  cos pi/2 : Constant  Value=[cos(-angle_roll/2)]
  sin pi/4 : Constant  Value=sin(-angle_roll/2)
  Q_rot : Outport  VectorParamsAs1DForOutWhenUnconnected=off
  wires:
  cos pi/2/1 -> Vector Concatenate1/1
  Vector Concatenate1/1 -> Q_rot/1
  sin pi/4/1 -> Product/2
  Product/1 -> Reshape1/1
  Reshape1/1 -> Vector Concatenate1/2
  Constant/1 -> Product/1  "x"

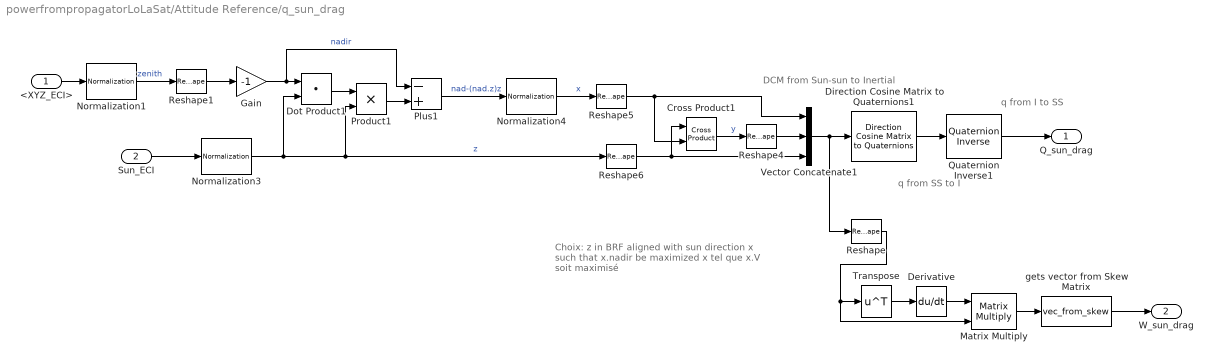
== system powerfrompropagatorLoLaSat/Attitude Reference/q_sun_drag ==
  note: Choix:
      | z in BRF aligned with sun direction
      | x such that x.nadir be maximized
      | x tel que x.V soit maximisé
  note: DCM from Sun-sun to Inertial
  note: q from I to SS
  note: q from SS to I
  <XYZ_ECI> : Inport
  Sun_ECI : Inport  Port=2
  Cross Product1 : vrlib/Utilities/Cross Product
  Derivative : Derivative
  Direction Cosine Matrix to Quaternions1 : sharedtransform/Direction Cosine Matrix  to Quaternions  aMode=0  action=None  tolerance=eps(2)
  Dot Product1 : DotProduct  OutDataTypeStr=Inherit: Inherit via internal rule
  Gain : Gain  Gain=-1
  Matrix Multiply : Product  Multiplication=Matrix(*)
  Normalization1 : dspmathops/Normalization  NormType=2-norm  Bias=1e-10  NormOver=Each column  Dimension=1  roundingMode=Floor  overflowMode=off  accumDataTypeStr=Inherit: Same as product output  accumLastDataTypeStr=Inherit: Same as product output  outputDataTypeStr=Inherit: Same as product output  outputMin=[]  outputMax=[]  outputLastDataTypeStr=Inherit: Same as product output
  Normalization3 : dspmathops/Normalization  NormType=2-norm  Bias=1e-10  NormOver=Each column  Dimension=1  roundingMode=Floor  overflowMode=off  accumDataTypeStr=Inherit: Same as product output  accumLastDataTypeStr=Inherit: Same as product output  outputDataTypeStr=Inherit: Same as product output  outputMin=[]  outputMax=[]  outputLastDataTypeStr=Inherit: Same as product output
  Normalization4 : dspmathops/Normalization  NormType=2-norm  Bias=1e-10  NormOver=Each column  Dimension=1  roundingMode=Floor  overflowMode=off  accumDataTypeStr=Inherit: Same as product output  accumLastDataTypeStr=Inherit: Same as product output  outputDataTypeStr=Inherit: Same as product output  outputMin=[]  outputMax=[]  outputLastDataTypeStr=Inherit: Same as product output
  Plus1 : Sum  Inputs=-+
  Product1 : Product
  Quaternion Inverse1 : aerolibutil/Quaternion Inverse
  Reshape : Reshape  OutputDimensionality=Customize  OutputDimensions=[3,3]
  Reshape{1,4..6} (4 alike) : Reshape  OutputDimensionality=Column vector (2-D)
  Transpose : Math  Operator=transpose
  Vector Concatenate1 : Concatenate  NumInputs=3  Mode=Multidimensional array  ConcatenateDimension=2
  gets vector from Skew Matrix : MATLABFcn  MATLABFcn=vec_from_skew
  Q_sun_drag : Outport  VectorParamsAs1DForOutWhenUnconnected=off
  W_sun_drag : Outport  Port=2
  wires:
  Direction Cosine Matrix to Quaternions1/1 -> Quaternion Inverse1/1
  Reshape4/1 -> Vector Concatenate1/2
  Dot Product1/1 -> Product1/1
  Sun_ECI/1 -> Normalization3/1
  Quaternion Inverse1/1 -> Q_sun_drag/1
  Reshape1/1 -> Gain/1
  Plus1/1 -> Normalization4/1  "nad-(nad.z)z"
  Reshape6/1 -> Cross Product1/1, Vector Concatenate1/3
  Normalization3/1 -> Dot Product1/2, Product1/2, Reshape6/1  "z"
  Reshape5/1 -> Cross Product1/2, Vector Concatenate1/1
  Cross Product1/1 -> Reshape4/1  "y"
  Normalization4/1 -> Reshape5/1  "x"
  Product1/1 -> Plus1/2
  Reshape/1 -> Matrix Multiply/2, Transpose/1
  Derivative/1 -> Matrix Multiply/1
  Transpose/1 -> Derivative/1
  Matrix Multiply/1 -> gets vector from Skew Matrix/1
  gets vector from Skew Matrix/1 -> W_sun_drag/1
  Vector Concatenate1/1 -> Direction Cosine Matrix to Quaternions1/1, Reshape/1
  <XYZ_ECI>/1 -> Normalization1/1
  Normalization1/1 -> Reshape1/1  "zenith"
  Gain/1 -> Dot Product1/1, Plus1/1  "nadir"

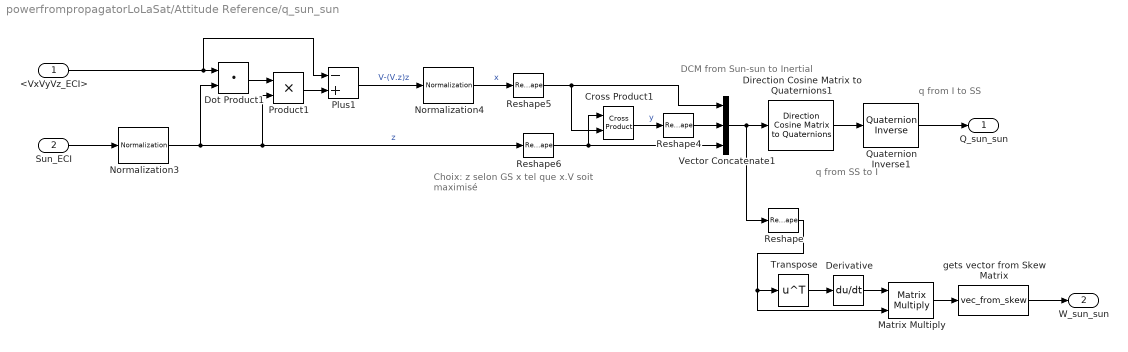
== system powerfrompropagatorLoLaSat/Attitude Reference/q_sun_sun ==
  note: Choix:
      | z selon GS
      | x tel que x.V soit maximisé
  note: DCM from Sun-sun to Inertial
  note: q from I to SS
  note: q from SS to I
  <VxVyVz_ECI> : Inport
  Sun_ECI : Inport  Port=2
  Cross Product1 : vrlib/Utilities/Cross Product
  Derivative : Derivative
  Direction Cosine Matrix to Quaternions1 : sharedtransform/Direction Cosine Matrix  to Quaternions  aMode=0  action=None  tolerance=eps(2)
  Dot Product1 : DotProduct  OutDataTypeStr=Inherit: Inherit via internal rule
  Matrix Multiply : Product  Multiplication=Matrix(*)
  Normalization3 : dspmathops/Normalization  NormType=2-norm  Bias=1e-10  NormOver=Each column  Dimension=1  roundingMode=Floor  overflowMode=off  accumDataTypeStr=Inherit: Same as product output  accumLastDataTypeStr=Inherit: Same as product output  outputDataTypeStr=Inherit: Same as product output  outputMin=[]  outputMax=[]  outputLastDataTypeStr=Inherit: Same as product output
  Normalization4 : dspmathops/Normalization  NormType=2-norm  Bias=1e-10  NormOver=Each column  Dimension=1  roundingMode=Floor  overflowMode=off  accumDataTypeStr=Inherit: Same as product output  accumLastDataTypeStr=Inherit: Same as product output  outputDataTypeStr=Inherit: Same as product output  outputMin=[]  outputMax=[]  outputLastDataTypeStr=Inherit: Same as product output
  Plus1 : Sum  Inputs=-+
  Product1 : Product
  Quaternion Inverse1 : aerolibutil/Quaternion Inverse
  Reshape : Reshape  OutputDimensionality=Customize  OutputDimensions=[3,3]
  Reshape4 : Reshape  OutputDimensionality=Column vector (2-D)
  Reshape5 : Reshape  OutputDimensionality=Column vector (2-D)
  Reshape6 : Reshape  OutputDimensionality=Column vector (2-D)
  Transpose : Math  Operator=transpose
  Vector Concatenate1 : Concatenate  NumInputs=3  Mode=Multidimensional array  ConcatenateDimension=2
  gets vector from Skew Matrix : MATLABFcn  MATLABFcn=vec_from_skew
  Q_sun_sun : Outport  VectorParamsAs1DForOutWhenUnconnected=off
  W_sun_sun : Outport  Port=2
  wires:
  Direction Cosine Matrix to Quaternions1/1 -> Quaternion Inverse1/1
  Reshape4/1 -> Vector Concatenate1/2
  Dot Product1/1 -> Product1/1
  Sun_ECI/1 -> Normalization3/1
  Quaternion Inverse1/1 -> Q_sun_sun/1
  <VxVyVz_ECI>/1 -> Dot Product1/1, Plus1/1
  Plus1/1 -> Normalization4/1  "V-(V.z)z"
  Reshape6/1 -> Cross Product1/1, Vector Concatenate1/3
  Normalization3/1 -> Dot Product1/2, Product1/2, Reshape6/1  "z"
  Reshape5/1 -> Cross Product1/2, Vector Concatenate1/1
  Cross Product1/1 -> Reshape4/1  "y"
  Normalization4/1 -> Reshape5/1  "x"
  Product1/1 -> Plus1/2
  Reshape/1 -> Matrix Multiply/2, Transpose/1
  Derivative/1 -> Matrix Multiply/1
  Transpose/1 -> Derivative/1
  Matrix Multiply/1 -> gets vector from Skew Matrix/1
  gets vector from Skew Matrix/1 -> W_sun_sun/1
  Vector Concatenate1/1 -> Direction Cosine Matrix to Quaternions1/1, Reshape/1

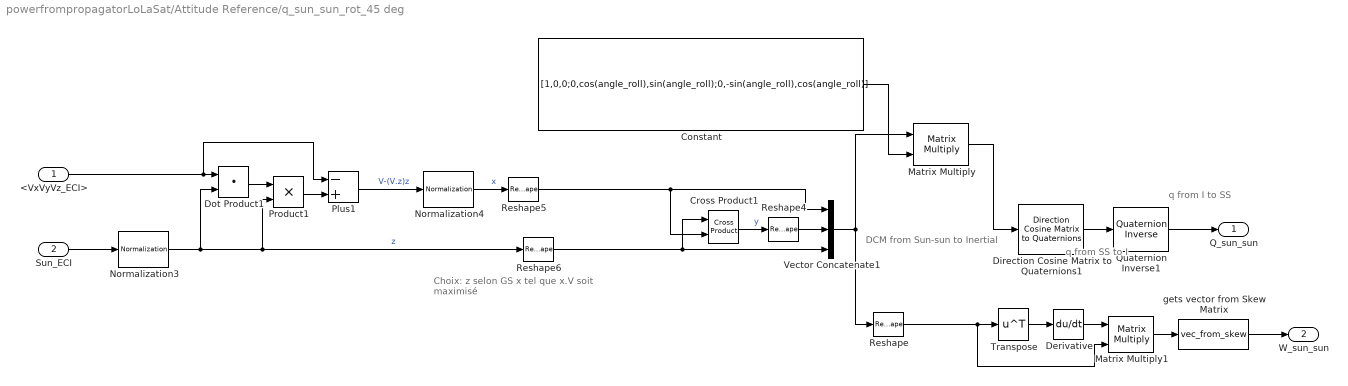
== system powerfrompropagatorLoLaSat/Attitude Reference/q_sun_sun_rot_45 deg ==
  note: Choix:
      | z selon GS
      | x tel que x.V soit maximisé
  note: DCM from Sun-sun to Inertial
  note: q from I to SS
  note: q from SS to I
  <VxVyVz_ECI> : Inport
  Sun_ECI : Inport  Port=2
  Constant : Constant  Value=[1,0,0;0,cos(angle_roll),sin(angle_roll);0,-sin(angle_roll),cos(angle_roll)]
  Cross Product1 : vrlib/Utilities/Cross Product
  Derivative : Derivative
  Direction Cosine Matrix to Quaternions1 : sharedtransform/Direction Cosine Matrix  to Quaternions  aMode=0  action=None  tolerance=eps(2)
  Dot Product1 : DotProduct  OutDataTypeStr=Inherit: Inherit via internal rule
  Matrix Multiply : Product  Multiplication=Matrix(*)
  Matrix Multiply1 : Product  Multiplication=Matrix(*)
  Normalization3 : dspmathops/Normalization  NormType=2-norm  Bias=1e-10  NormOver=Each column  Dimension=1  roundingMode=Floor  overflowMode=off  accumDataTypeStr=Inherit: Same as product output  accumLastDataTypeStr=Inherit: Same as product output  outputDataTypeStr=Inherit: Same as product output  outputMin=[]  outputMax=[]  outputLastDataTypeStr=Inherit: Same as product output
  Normalization4 : dspmathops/Normalization  NormType=2-norm  Bias=1e-10  NormOver=Each column  Dimension=1  roundingMode=Floor  overflowMode=off  accumDataTypeStr=Inherit: Same as product output  accumLastDataTypeStr=Inherit: Same as product output  outputDataTypeStr=Inherit: Same as product output  outputMin=[]  outputMax=[]  outputLastDataTypeStr=Inherit: Same as product output
  Plus1 : Sum  Inputs=-+
  Product1 : Product
  Quaternion Inverse1 : aerolibutil/Quaternion Inverse
  Reshape : Reshape  OutputDimensionality=Customize  OutputDimensions=[3,3]
  Reshape4 : Reshape  OutputDimensionality=Column vector (2-D)
  Reshape5 : Reshape  OutputDimensionality=Column vector (2-D)
  Reshape6 : Reshape  OutputDimensionality=Column vector (2-D)
  Transpose : Math  Operator=transpose
  Vector Concatenate1 : Concatenate  NumInputs=3  Mode=Multidimensional array  ConcatenateDimension=2
  gets vector from Skew Matrix : MATLABFcn  MATLABFcn=vec_from_skew
  Q_sun_sun : Outport  VectorParamsAs1DForOutWhenUnconnected=off
  W_sun_sun : Outport  Port=2
  wires:
  Reshape4/1 -> Vector Concatenate1/2
  Dot Product1/1 -> Product1/1
  Sun_ECI/1 -> Normalization3/1
  Quaternion Inverse1/1 -> Q_sun_sun/1
  <VxVyVz_ECI>/1 -> Dot Product1/1, Plus1/1
  Plus1/1 -> Normalization4/1  "V-(V.z)z"
  Reshape6/1 -> Cross Product1/1, Vector Concatenate1/3
  Normalization3/1 -> Dot Product1/2, Product1/2, Reshape6/1  "z"
  Reshape5/1 -> Cross Product1/2, Vector Concatenate1/1
  Cross Product1/1 -> Reshape4/1  "y"
  Normalization4/1 -> Reshape5/1  "x"
  Product1/1 -> Plus1/2
  Direction Cosine Matrix to Quaternions1/1 -> Quaternion Inverse1/1
  Constant/1 -> Matrix Multiply/2
  Vector Concatenate1/1 -> Matrix Multiply/1, Reshape/1
  Matrix Multiply/1 -> Direction Cosine Matrix to Quaternions1/1
  Transpose/1 -> Derivative/1
  gets vector from Skew Matrix/1 -> W_sun_sun/1
  Reshape/1 -> Matrix Multiply1/2, Transpose/1
  Derivative/1 -> Matrix Multiply1/1
  Matrix Multiply1/1 -> gets vector from Skew Matrix/1

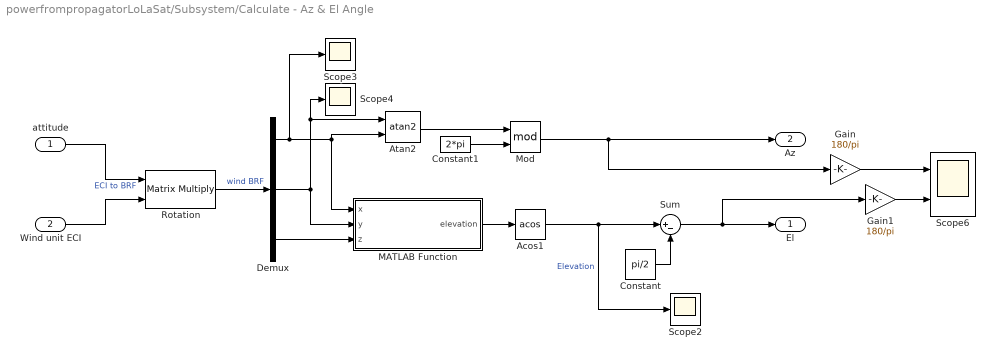
== system powerfrompropagatorLoLaSat/Subsystem/Calculate - Az & El Angle ==
  attitude : Inport
  Wind unit ECI : Inport  Port=2
  Acos1 : Trigonometry  Operator=acos
  Atan2 : Trigonometry  Operator=atan2
  Constant : Constant  Value=pi/2
  Constant1 : Constant  Value=2*pi
  Demux : Demux  Outputs=3
  Gain : Gain  Gain=180/pi
  Gain1 : Gain  Gain=180/pi
  MATLAB Function : MATLAB Function  TreatAsAtomicUnit=on
  Mod : Math  Operator=mod  OutMin=[0]  OutMax=[2*pi]
  Rotation : Product  Multiplication=Matrix(*)  RndMeth=Zero
  Scope2 : Scope
  Scope3 : Scope
  Scope4 : Scope
  Scope6 : Scope  NumInputPorts=2
  Sum : Sum  Inputs=|+-
  El : Outport
  Az : Outport  Port=2
  wires:
  attitude/1 -> Rotation/1  "ECI to BRF"
  Wind unit ECI/1 -> Rotation/2
  Mod/1 -> Gain/1, Az/1
  Constant1/1 -> Mod/2
  Atan2/1 -> Mod/1
  MATLAB Function/1(elevation) -> Acos1/1
  Sum/1 -> Gain1/1, El/1
  Acos1/1 -> Scope2/1, Sum/1  "Elevation"
  Demux/3 -> MATLAB Function/3(z)
  Rotation/1 -> Demux/1  "wind BRF"
  Demux/2 -> MATLAB Function/2(y), Scope4/1, Atan2/1
  Constant/1 -> Sum/2
  Demux/1 -> Atan2/2, MATLAB Function/1(x), Scope3/1
  Gain/1 -> Scope6/1
  Gain1/1 -> Scope6/2

== matlab function powerfrompropagatorLoLaSat/Subsystem/Calculate - Az & El Angle/MATLAB Function ==
  data: x input; elevation output; y input; z input
function elevation = fcn(x,y,z)

elevation = z/sqrt(x^2 + y^2 + z^2);
